simulink model "exm2_2"  (Simulink 3.00)
settings: Solver=VariableStepDiscrete  SolverMode=SingleTasking  StartTime=0.0  StopTime=10.0  RelTol=1e-3  AbsTol=1e-6
settings Model: RTWTemplateMakefile=grt_vc.tmf

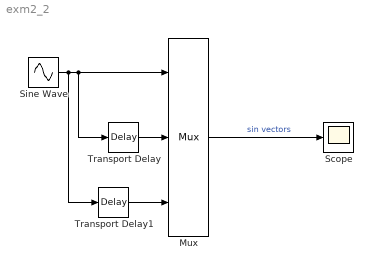
== system exm2_2 ==
  Mux : Mux  Inputs=3
      settings: DisplayOption=none
  Scope : Scope
      settings: TickLabels=on  TimeRange=10  YMin=-2  YMax=2  SaveToWorkspace=off  SaveName=ScopeData  DataFormat=Matrix
  Sine Wave : Sin  Amplitude=1  Frequency=1  Phase=0  SampleTime=0
  Transport Delay : TransportDelay  DelayTime=1  InitialInput=0  BufferSize=1024
  Transport Delay1 : TransportDelay  DelayTime=2  InitialInput=0  BufferSize=1024
  wires:
  Transport Delay/1 -> Mux/2
  Transport Delay1/1 -> Mux/3
  Sine Wave/1 -> Mux/1, Transport Delay/1, Transport Delay1/1
  Mux/1 -> Scope/1  "sin vectors"
